simulink model "Demo1System"  (R2022b)
settings: Solver=VariableStepAuto  StartTime=0.0  StopTime=40  RelTol=1e-3
values from neighbouring files (symbols this model uses):
  b = .5    (= 0.5)    [RunDemo1System.m]    (also in RunDemo1SystemNoCamera.m)
  d = 28 * ft_per_cm    (= 0.9186352)    [RunDemo1System.m]    (also in RunDemo1SystemNoCamera.m)
  J = .05    (= 0.05)    [RunDemo1System.m]    (also in RunDemo1SystemNoCamera.m)
  Ke = .5    (= 0.5)    [RunDemo1System.m]    (also in RunDemo1SystemNoCamera.m)
  Kt = .5    (= 0.5)    [RunDemo1System.m]    (also in RunDemo1SystemNoCamera.m)
  r = 7.5 * ft_per_cm    (= 0.246063)    [RunDemo1System.m]    (also in RunDemo1SystemNoCamera.m)
  Ra = 1    [RunDemo1System.m]    (also in RunDemo1SystemNoCamera.m)
  rho_dot_des = 0.2    [RunDemo1System.m]    (also in RunDemo1SystemNoCamera.m = 0.5)
  xs = [0 3 6 10]    [RunDemo1System.m]
  ys = [0 0 3 3]    [RunDemo1System.m]
libraries: slpidlib x3
settings Model: Creator=Dawson  LastModifiedBy=Dawson

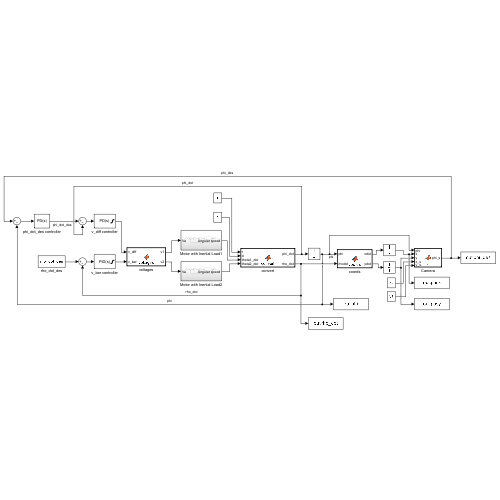
[thumbnail: Simulink's stored preview of the top-level diagram]
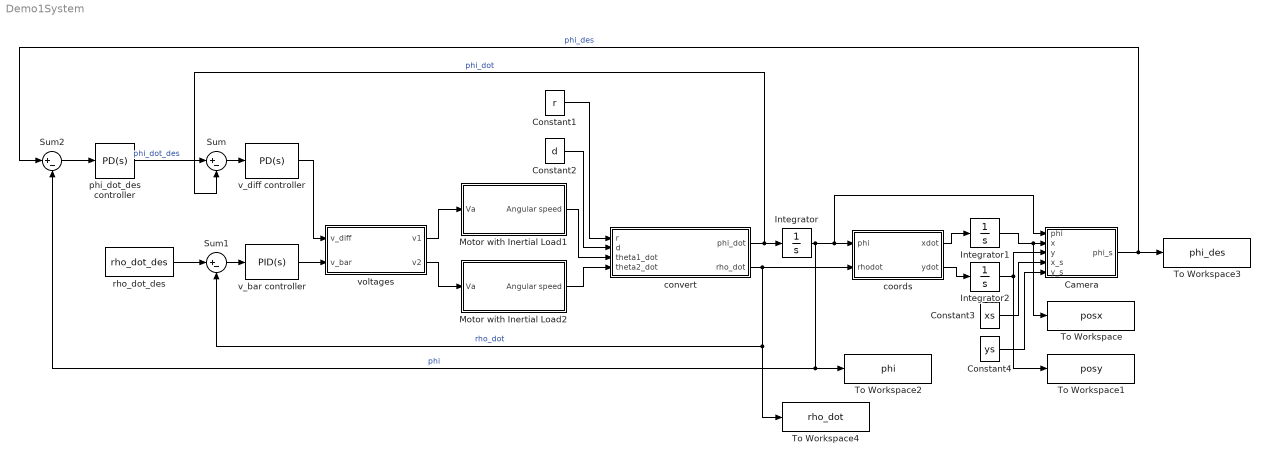
== system Demo1System ==
  Camera : MATLAB Function  TreatAsAtomicUnit=on  SystemSampleTime=.2
  Constant1 : Constant  Value=r
  Constant2 : Constant  Value=d
  Constant3 : Constant  Value=xs
  Constant4 : Constant  Value=ys
  Integrator : Integrator
  Integrator1 : Integrator
  Integrator2 : Integrator
  Motor with Inertial Load1 : Subsystem
  Motor with Inertial Load2 : Subsystem
  Sum : Sum  Inputs=|+-
  Sum1 : Sum  Inputs=|+-
  Sum2 : Sum  Inputs=|+-
  To Workspace : ToWorkspace  VariableName=posx  SaveFormat=Timeseries  SampleTime=-1
  To Workspace1 : ToWorkspace  VariableName=posy  SaveFormat=Timeseries  SampleTime=-1
  To Workspace2 : ToWorkspace  VariableName=phi  SaveFormat=Timeseries  SampleTime=-1
  To Workspace3 : ToWorkspace  VariableName=phi_des  SaveFormat=Timeseries  SampleTime=-1
  To Workspace4 : ToWorkspace  VariableName=rho_dot  SaveFormat=Timeseries  SampleTime=-1
  convert : MATLAB Function  TreatAsAtomicUnit=on
  coords : MATLAB Function  TreatAsAtomicUnit=on
  phi_dot_des controller : slpidlib/PID Controller  Controller=PD  Form=Parallel  TimeDomain=Continuous-time  UseExternalTs=off  SampleTime=-1  IntegratorMethod=Forward Euler  FilterMethod=Forward Euler  ControllerParametersSource=internal  P=10.0051896084746  I=0.00593939817102329  UseKiTs=off  D=0.000344949119801465  N=5045.83326424297  UseFilter=on  TunerSelectOption=Transfer Function Based (PID Tuner App)  InitialConditionSource=internal  InitialConditionForIntegrator=0  InitialConditionForFilter=0  DifferentiatorICPrevScaledInput=0  ExternalReset=none  TrackingMode=off  Kt=1  LimitOutput=off  SatLimitsSource=internal  UpperSaturationLimit=inf  LowerSaturationLimit=-inf  LinearizeAsGain=on  AntiWindupMode=none  Kb=1  LimitIntegrator=off  UpperIntegratorSaturationLimit=inf  LowerIntegratorSaturationLimit=-inf  POutMin=[]  POutMax=[]  IOutMin=[]  IOutMax=[]  DOutMin=[]  DOutMax=[]  NOutMin=[]  NOutMax=[]  SumOutMin=[]  SumOutMax=[]  SaturationOutMin=[]  SaturationOutMax=[]  PParamMin=[]  PParamMax=[]  IParamMin=[]  IParamMax=[]  DParamMin=[]  DParamMax=[]  NParamMin=[]  NParamMax=[]  KbParamMin=[]  KbParamMax=[]  KtParamMin=[]  KtParamMax=[]  KbOutMin=[]  KbOutMax=[]  KtOutMin=[]  KtOutMax=[]  IntegratorOutMin=[]  IntegratorOutMax=[]  FilterOutMin=[]  FilterOutMax=[]  SumI1OutMin=[]  SumI1OutMax=[]  SumI2OutMin=[]  SumI2OutMax=[]  SumI3OutMin=[]  SumI3OutMax=[]  SumI4OutMin=[]  SumI4OutMax=[]  SumDOutMin=[]  SumDOutMax=[]  DifferentiatorOutMin=[]  DifferentiatorOutMax=[]  FilterDiffOutCoefMin=[]  FilterDiffOutCoefMax=[]  ReciprocalOutMin=[]  ReciprocalOutMax=[]  SumDenOutMin=[]  SumDenOutMax=[]  SumNumOutMin=[]  SumNumOutMax=[]  DivideOutMin=[]  DivideOutMax=[]  UdiffTsProdOutMin=[]  UdiffTsProdOutMax=[]  NTsProdOutMin=[]  NTsProdOutMax=[]  UintegralTsProdOutMin=[]  UintegralTsProdOutMax=[]  UngainTsProdOutMin=[]  UngainTsProdOutMax=[]  ClampingZeroOutDataTypeStr=Inherit: Inherit via back propagation  ClampingZeroOutMin=[]  ClampingZeroOutMax=[]  FilterDenConstantOutDataTypeStr=Inherit: Inherit via back propagation  FilterDenConstantOutMin=[]  FilterDenConstantOutMax=[]  PCopyOutDataTypeStr=Inherit: Inherit via back propagation  PCopyOutMin=[]  PCopyOutMax=[]  NCopyOutDataTypeStr=Inherit: Inherit via back propagation  NCopyOutMin=[]  NCopyOutMax=[]  IntegratorContinuousStateAttributes=''  IntegratorStateMustResolveToSignalObject=off  IntegratorRTWStateStorageClass=Auto  FilterContinuousStateAttributes=''  FilterStateMustResolveToSignalObject=off  FilterRTWStateStorageClass=Auto  ParallelPVariant=InternalParameters  IdealPVariant=Disabled  IVariant=Disabled  DVariant=InternalParameters  IntegratorVariant=Disabled  SatVariant=Disabled  AWVariant=Disabled  PCopyVariant=Disabled  TRVariant=Disabled  FdbkBlocksVariant=Forward  IdealPFdbkVariant=Disabled  SatFdbkVariant=Disabled  DerivativeFilterVariant=ContFilter  NVariant=InternalParameters  NCopyVariant=Disabled  FilterICVariant=InternalICsFilter  IntegratorICVariant=Disabled  ExternalResetVariant=Disabled  TRSumVariant=Passthrough  SumFdbkVariant=Disabled  SumVariant=Sum_PD  TsampFilterVariant=InternalTs  TsampNgainVariant=Passthrough  TsampIntegralVariant=Disabled_SignalSpec  ExternalSaturationOutDataTypeStr=Inherit: Same as second input
  rho_dot_des : Constant  Value=rho_dot_des
  v_bar controller : slpidlib/PID Controller  Controller=PID  Form=Parallel  TimeDomain=Continuous-time  UseExternalTs=off  SampleTime=-1  IntegratorMethod=Forward Euler  FilterMethod=Forward Euler  ControllerParametersSource=internal  P=7.14216735267938  I=119.884076500748  UseKiTs=off  D=-0.0950863513693689  N=7138830.05741258  UseFilter=on  TunerSelectOption=Transfer Function Based (PID Tuner App)  InitialConditionSource=internal  InitialConditionForIntegrator=0  InitialConditionForFilter=0  DifferentiatorICPrevScaledInput=0  ExternalReset=none  TrackingMode=off  Kt=1  LimitOutput=on  SatLimitsSource=internal  UpperSaturationLimit=7.8  LowerSaturationLimit=-7.8  LinearizeAsGain=on  AntiWindupMode=none  Kb=1  LimitIntegrator=off  UpperIntegratorSaturationLimit=inf  LowerIntegratorSaturationLimit=-inf  POutMin=[]  POutMax=[]  IOutMin=[]  IOutMax=[]  DOutMin=[]  DOutMax=[]  NOutMin=[]  NOutMax=[]  SumOutMin=[]  SumOutMax=[]  SaturationOutMin=[]  SaturationOutMax=[]  PParamMin=[]  PParamMax=[]  IParamMin=[]  IParamMax=[]  DParamMin=[]  DParamMax=[]  NParamMin=[]  NParamMax=[]  KbParamMin=[]  KbParamMax=[]  KtParamMin=[]  KtParamMax=[]  KbOutMin=[]  KbOutMax=[]  KtOutMin=[]  KtOutMax=[]  IntegratorOutMin=[]  IntegratorOutMax=[]  FilterOutMin=[]  FilterOutMax=[]  SumI1OutMin=[]  SumI1OutMax=[]  SumI2OutMin=[]  SumI2OutMax=[]  SumI3OutMin=[]  SumI3OutMax=[]  SumI4OutMin=[]  SumI4OutMax=[]  SumDOutMin=[]  SumDOutMax=[]  DifferentiatorOutMin=[]  DifferentiatorOutMax=[]  FilterDiffOutCoefMin=[]  FilterDiffOutCoefMax=[]  ReciprocalOutMin=[]  ReciprocalOutMax=[]  SumDenOutMin=[]  SumDenOutMax=[]  SumNumOutMin=[]  SumNumOutMax=[]  DivideOutMin=[]  DivideOutMax=[]  UdiffTsProdOutMin=[]  UdiffTsProdOutMax=[]  NTsProdOutMin=[]  NTsProdOutMax=[]  UintegralTsProdOutMin=[]  UintegralTsProdOutMax=[]  UngainTsProdOutMin=[]  UngainTsProdOutMax=[]  ClampingZeroOutDataTypeStr=Inherit: Inherit via back propagation  ClampingZeroOutMin=[]  ClampingZeroOutMax=[]  FilterDenConstantOutDataTypeStr=Inherit: Inherit via back propagation  FilterDenConstantOutMin=[]  FilterDenConstantOutMax=[]  PCopyOutDataTypeStr=Inherit: Inherit via back propagation  PCopyOutMin=[]  PCopyOutMax=[]  NCopyOutDataTypeStr=Inherit: Inherit via back propagation  NCopyOutMin=[]  NCopyOutMax=[]  IntegratorContinuousStateAttributes=''  IntegratorStateMustResolveToSignalObject=off  IntegratorRTWStateStorageClass=Auto  FilterContinuousStateAttributes=''  FilterStateMustResolveToSignalObject=off  FilterRTWStateStorageClass=Auto  ParallelPVariant=InternalParameters  IdealPVariant=Disabled  IVariant=InternalParameters  DVariant=InternalParameters  IntegratorVariant=Continuous  SatVariant=Enabled  AWVariant=Passthrough  PCopyVariant=Disabled  TRVariant=Disabled  FdbkBlocksVariant=Forward  IdealPFdbkVariant=Disabled  SatFdbkVariant=Disabled  DerivativeFilterVariant=ContFilter  NVariant=InternalParameters  NCopyVariant=Disabled  FilterICVariant=InternalICsFilter  IntegratorICVariant=InternalICs  ExternalResetVariant=Disabled  TRSumVariant=Passthrough  SumFdbkVariant=Disabled  SumVariant=Sum_PID  TsampFilterVariant=InternalTs  TsampNgainVariant=Passthrough  TsampIntegralVariant=Passthrough  ExternalSaturationOutDataTypeStr=Inherit: Same as second input
  v_diff controller : slpidlib/PID Controller  Controller=PD  Form=Parallel  TimeDomain=Continuous-time  UseExternalTs=off  SampleTime=-1  IntegratorMethod=Forward Euler  FilterMethod=Forward Euler  ControllerParametersSource=internal  P=10791.2170261385  I=63.6988918390083  UseKiTs=off  D=2.15324649932964  N=24307.6852720481  UseFilter=on  TunerSelectOption=Transfer Function Based (PID Tuner App)  InitialConditionSource=internal  InitialConditionForIntegrator=0  InitialConditionForFilter=0  DifferentiatorICPrevScaledInput=0  ExternalReset=none  TrackingMode=off  Kt=1  LimitOutput=on  SatLimitsSource=internal  UpperSaturationLimit=7.8  LowerSaturationLimit=-7.8  LinearizeAsGain=on  AntiWindupMode=none  Kb=1  LimitIntegrator=off  UpperIntegratorSaturationLimit=inf  LowerIntegratorSaturationLimit=-inf  POutMin=[]  POutMax=[]  IOutMin=[]  IOutMax=[]  DOutMin=[]  DOutMax=[]  NOutMin=[]  NOutMax=[]  SumOutMin=[]  SumOutMax=[]  SaturationOutMin=[]  SaturationOutMax=[]  PParamMin=[]  PParamMax=[]  IParamMin=[]  IParamMax=[]  DParamMin=[]  DParamMax=[]  NParamMin=[]  NParamMax=[]  KbParamMin=[]  KbParamMax=[]  KtParamMin=[]  KtParamMax=[]  KbOutMin=[]  KbOutMax=[]  KtOutMin=[]  KtOutMax=[]  IntegratorOutMin=[]  IntegratorOutMax=[]  FilterOutMin=[]  FilterOutMax=[]  SumI1OutMin=[]  SumI1OutMax=[]  SumI2OutMin=[]  SumI2OutMax=[]  SumI3OutMin=[]  SumI3OutMax=[]  SumI4OutMin=[]  SumI4OutMax=[]  SumDOutMin=[]  SumDOutMax=[]  DifferentiatorOutMin=[]  DifferentiatorOutMax=[]  FilterDiffOutCoefMin=[]  FilterDiffOutCoefMax=[]  ReciprocalOutMin=[]  ReciprocalOutMax=[]  SumDenOutMin=[]  SumDenOutMax=[]  SumNumOutMin=[]  SumNumOutMax=[]  DivideOutMin=[]  DivideOutMax=[]  UdiffTsProdOutMin=[]  UdiffTsProdOutMax=[]  NTsProdOutMin=[]  NTsProdOutMax=[]  UintegralTsProdOutMin=[]  UintegralTsProdOutMax=[]  UngainTsProdOutMin=[]  UngainTsProdOutMax=[]  ClampingZeroOutDataTypeStr=Inherit: Inherit via back propagation  ClampingZeroOutMin=[]  ClampingZeroOutMax=[]  FilterDenConstantOutDataTypeStr=Inherit: Inherit via back propagation  FilterDenConstantOutMin=[]  FilterDenConstantOutMax=[]  PCopyOutDataTypeStr=Inherit: Inherit via back propagation  PCopyOutMin=[]  PCopyOutMax=[]  NCopyOutDataTypeStr=Inherit: Inherit via back propagation  NCopyOutMin=[]  NCopyOutMax=[]  IntegratorContinuousStateAttributes=''  IntegratorStateMustResolveToSignalObject=off  IntegratorRTWStateStorageClass=Auto  FilterContinuousStateAttributes=''  FilterStateMustResolveToSignalObject=off  FilterRTWStateStorageClass=Auto  ParallelPVariant=InternalParameters  IdealPVariant=Disabled  IVariant=Disabled  DVariant=InternalParameters  IntegratorVariant=Disabled  SatVariant=Enabled  AWVariant=Disabled  PCopyVariant=Disabled  TRVariant=Disabled  FdbkBlocksVariant=Forward  IdealPFdbkVariant=Disabled  SatFdbkVariant=Disabled  DerivativeFilterVariant=ContFilter  NVariant=InternalParameters  NCopyVariant=Disabled  FilterICVariant=InternalICsFilter  IntegratorICVariant=Disabled  ExternalResetVariant=Disabled  TRSumVariant=Passthrough  SumFdbkVariant=Disabled  SumVariant=Sum_PD  TsampFilterVariant=InternalTs  TsampNgainVariant=Passthrough  TsampIntegralVariant=Disabled_SignalSpec  ExternalSaturationOutDataTypeStr=Inherit: Same as second input
  voltages : MATLAB Function  TreatAsAtomicUnit=on
  wires:
  Sum/1 -> v_diff controller/1
  Sum1/1 -> v_bar controller/1
  Sum2/1 -> phi_dot_des controller/1
  phi_dot_des controller/1 -> Sum/1  "phi_dot_des"
  v_diff controller/1 -> voltages/1(v_diff)
  v_bar controller/1 -> voltages/2(v_bar)
  voltages/1(v1) -> Motor with Inertial Load1/1(Va)
  rho_dot_des/1 -> Sum1/1
  voltages/2(v2) -> Motor with Inertial Load2/1(Va)
  Motor with Inertial Load1/1(Angular speed) -> convert/3(theta1_dot)
  Motor with Inertial Load2/1(Angular speed) -> convert/4(theta2_dot)
  Constant2/1 -> convert/2(d)
  Constant1/1 -> convert/1(r)
  Integrator/1 -> Sum2/2, To Workspace2/1, coords/1(phi), Camera/1(phi)  "phi"
  convert/2(rho_dot) -> To Workspace4/1, Sum1/2, coords/2(rhodot)  "rho_dot"
  coords/1(xdot) -> Integrator1/1
  coords/2(ydot) -> Integrator2/1
  Integrator2/1 -> Camera/3(y), To Workspace1/1
  Integrator1/1 -> To Workspace/1, Camera/2(x)
  Constant3/1 -> Camera/4(x_s)
  Constant4/1 -> Camera/5(y_s)
  Camera/1(phi_s) -> To Workspace3/1, Sum2/1  "phi_des"
  convert/1(phi_dot) -> Sum/2, Integrator/1  "phi_dot"

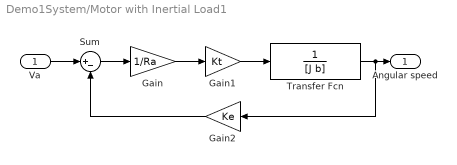
== system Demo1System/Motor with Inertial Load1 ==
  Va : Inport
  Gain : Gain  Gain=1/Ra
  Gain1 : Gain  Gain=Kt
  Gain2 : Gain  Gain=Ke
  Sum : Sum  Inputs=|+-
  Transfer Fcn : TransferFcn  Denominator=[J b]
  Angular speed : Outport
  wires:
  Gain/1 -> Gain1/1
  Transfer Fcn/1 -> Angular speed/1, Gain2/1
  Va/1 -> Sum/1
  Sum/1 -> Gain/1
  Gain1/1 -> Transfer Fcn/1
  Gain2/1 -> Sum/2

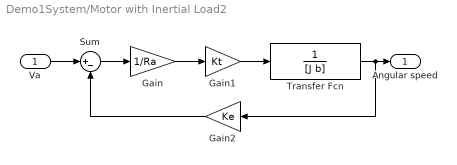
== system Demo1System/Motor with Inertial Load2 ==
  Va : Inport
  Gain : Gain  Gain=1/Ra
  Gain1 : Gain  Gain=Kt
  Gain2 : Gain  Gain=Ke
  Sum : Sum  Inputs=|+-
  Transfer Fcn : TransferFcn  Denominator=[J b]
  Angular speed : Outport
  wires:
  Gain/1 -> Gain1/1
  Transfer Fcn/1 -> Angular speed/1, Gain2/1
  Va/1 -> Sum/1
  Sum/1 -> Gain/1
  Gain1/1 -> Transfer Fcn/1
  Gain2/1 -> Sum/2

== matlab function Demo1System/coords ==
  data: phi input; xdot output; rhodot input; ydot output
function [xdot,ydot]= coords(phi,rhodot)
    xdot=rhodot*cos(phi);
    ydot=rhodot*sin(phi);
end

== matlab function Demo1System/Camera ==
  data: phi input; phi_s output; x input; y input; x_s input; y_s input
function phi_s = fcn(phi,x,y,x_s,y_s)
%#codegen
%
% Simulation of Camera with line detection
% phi - angle of robot in degrees
% x - x position of robot in feet
% y - y position of robot in feet
% x_s - vector of x coordinates for line to be detected (in feet)
% y_s - vector of y coordinates for line to be detected (in feet)
%
%

% change show_image to 1 to see camera image during simulation
show_image=1;
%
% number of horizontal and vertical pixels
%
h_pix = 740;
v_pix = 480;
%
% pixel_check is the row of the image to check for the line (origin of
% camera image is upper right
% 
pixel_check = v_pix*4/5;
%
% meters to feet conversion
%
mtof = 3.28;
% f is focal length 
%
f = .0036; %m
f = mtof*f; % convert to feet
%
% sensor image area
%
image_w = .00376; % m
image_h = .00274; % m
image_w = image_w*mtof; % convert to feet
image_h = image_h*mtof; % convert to feet
%
% h is height of the camera 
%
h = 0.1; % m
h = h*mtof; % convert to feet
%
% angle of view is from center to edge of camrea in radians
%
angle_of_view=53.5; % degrees

%
% interpolate between line points
%
x_s = interp1q((1:length(x_s))',x_s,(1:.01:length(x_s))');
y_s = interp1q((1:length(y_s))',y_s,(1:.01:length(y_s))');
%
% translate points to camera origin
% 
tape=[x_s,y_s]';
% figure
% plot(tape(1,:),tape(2,:),'*')
% axis([-5 5 -5 5])

tape = tape - [x;y]*ones(1,size(tape,2));
% figure
% plot(tape(1,:),tape(2,:),'*')
% axis([-5 5 -5 5])
%
% find points that are in the angle of view
%
angle = (180/pi)*acos(([cos(phi*pi/180) sin(phi*pi/180)]*tape)./sqrt(sum(tape.^2)));
index=find(angle<angle_of_view/2 & angle>-angle_of_view/2);
if isempty(index)
    disp('Tape not visible to the robot')
    phi_s = 0;
    return
end;
tape=tape(:,index);
% figure
% plot(tape(1,:),tape(2,:),'*')
% hold on
% fill(v_c(1,:),v_c(2,:),'y')
% title('visible points')
% axis([-5 5 -5 5])
%
% rotate points so straight ahead is along x axis
%
tapenorm=[cos(phi*pi/180) sin(phi*pi/180);-sin(phi*pi/180) cos(phi*pi/180)]*tape;
%
% map onto film coordinates
%
image = [(f./tapenorm(1,:)).*(-tapenorm(2,:));
    (f./tapenorm(1,:)).*(-h*ones(1,size(tapenorm,2)))];
% figure
% plot(image(1,:),image(2,:),'*')
% axis([-image_w/2 image_w/2 -image_h/2 image_h/2])

%
% map onto pixel coordinates
%
pixel = [0; v_pix]*ones(1,size(image,2)) + diag([h_pix/image_w -v_pix/image_h])*image+[h_pix/2; -v_pix/2]*ones(1,size(image,2));
if (show_image)
 figure(1)
 plot(pixel(1,:),pixel(2,:),'*')
 set(gca, 'YDir','reverse')
 hold on
 plot([0 h_pix],[pixel_check pixel_check],'r-')
 axis([0 h_pix 0 v_pix])
 hold off
 title('Robot camera view set show_image=0 to turn off and speed up simulation','interpreter','none')
end;


%
% find point on horizontal line at pixel number pixel_check
%
checkpoints= find(pixel(2,:)>=pixel_check);
if ~isempty(checkpoints)
    [m,index]=min(pixel(2,checkpoints));  
    if abs(pixel(2,index)-pixel_check)>10,
        disp(['no point visible near row ',int2str(pixel_check)])
        phi_s = 0;
        return
    end;
else
    disp(['no point visible near row ',int2str(pixel_check)])
    phi_s = 0;
    return
end;


phi_s = -(pixel(1,index)-h_pix/2)*angle_of_view/h_pix;

== matlab function Demo1System/voltages ==
  data: v_diff input; v1 output; v_bar input; v2 output
function [v1, v2] = voltages(v_diff, v_bar)
    v1 = (v_bar + v_diff)/2;
    v2 = (v_bar - v_diff)/2;
end

== matlab function Demo1System/convert ==
  data: r input; phi_dot output; d input; theta1_dot input; theta2_dot input; rho_dot output
function [phi_dot, rho_dot] = convert(r, d, theta1_dot, theta2_dot)
    phi_dot = (theta1_dot - theta2_dot)*r/d;
    rho_dot = (theta1_dot + theta2_dot)*r/2;
end
